simulink model "Dynamic_RLC_system_discrete"  (R2024a)
settings: Solver=FixedStepDiscrete  StartTime=0.0  StopTime=10.0  FixedStep=1e-3  MaxStep=1e-3  RelTol=1e-3
libraries: simulink x1
settings Model: Creator=DELL  LastModifiedBy=DELL

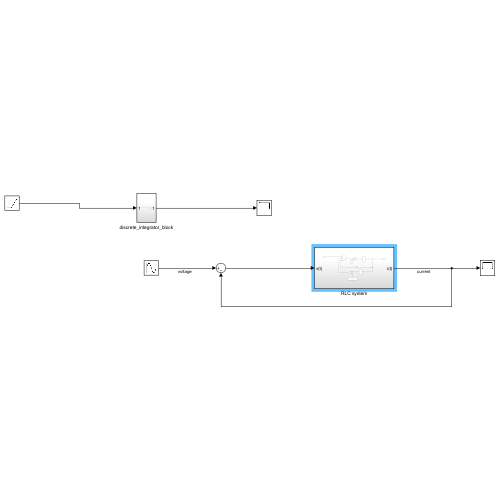
[thumbnail: Simulink's stored preview of the top-level diagram]
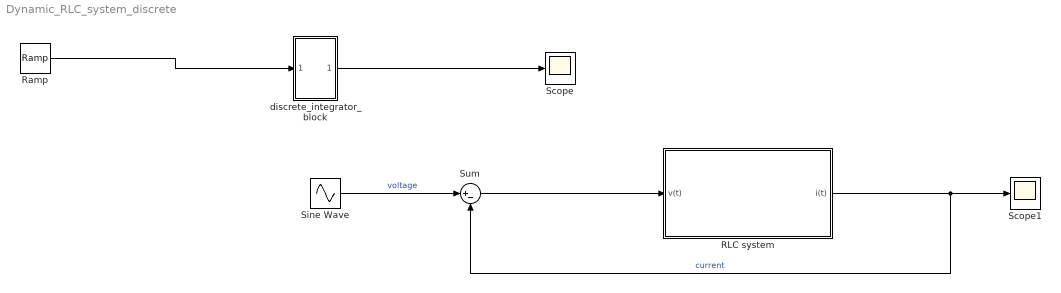
== system Dynamic_RLC_system_discrete ==
  RLC system : Subsystem
  Ramp : simulink/Sources/Ramp  slope=1  start=0  InitialOutput=0
  Scope : Scope
  Scope1 : Scope
  Sine Wave : Sin  Frequency=2000  SampleTime=0
  Sum : Sum  Inputs=|+-
  discrete_integrator_block : Subsystem
  wires:
  Ramp/1 -> discrete_integrator_block/1(In1)
  discrete_integrator_block/1(Out1) -> Scope/1
  Sum/1 -> RLC system/1(v(t))
  Sine Wave/1 -> Sum/1  "voltage"
  RLC system/1(i(t)) -> Sum/2, Scope1/1  "current"

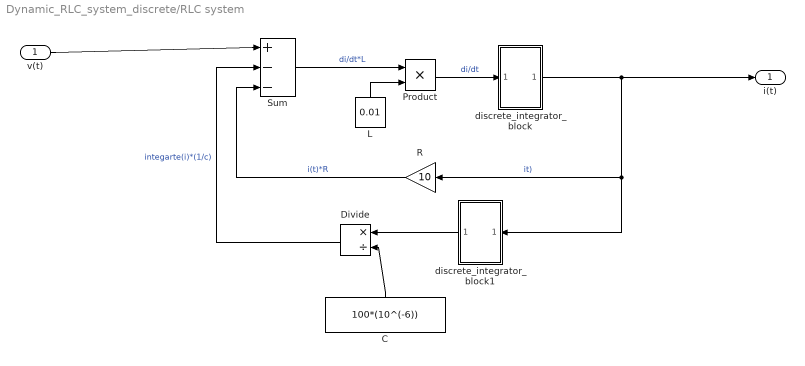
== system Dynamic_RLC_system_discrete/RLC system ==
  v(t) : Inport
  C : Constant  Value=100*(10^(-6))
  Divide : Product  Inputs=*/
  L : Constant  Value=0.01
  Product : Product
  R : Gain  Gain=10
  Sum : Sum  Inputs=|+|-|-
  discrete_integrator_block : Subsystem
  discrete_integrator_block1 : Subsystem
  i(t) : Outport
  wires:
  C/1 -> Divide/2
  L/1 -> Product/2
  discrete_integrator_block/1(Out1) -> i(t)/1, discrete_integrator_block1/1(In1), R/1  "it)"
  Divide/1 -> Sum/2  "integarte(i)*(1/c)"
  discrete_integrator_block1/1(Out1) -> Divide/1
  Product/1 -> discrete_integrator_block/1(In1)  "di/dt"
  Sum/1 -> Product/1  "di/dt*L"
  R/1 -> Sum/3  "i(t)*R"
  v(t)/1 -> Sum/1

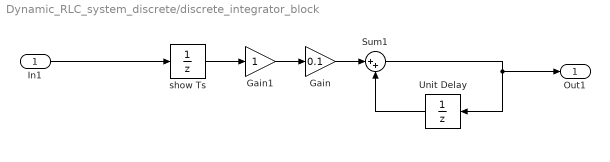
== system Dynamic_RLC_system_discrete/discrete_integrator_block ==
  In1 : Inport
  Gain : Gain  Gain=0.1
  Gain1 : Gain
  Sum1 : Sum  Inputs=|++
  Unit Delay : UnitDelay  SampleTime=-1  HasFrameUpgradeWarning=on
  show Ts : UnitDelay  SampleTime=-1  HasFrameUpgradeWarning=on
  Out1 : Outport
  wires:
  Gain1/1 -> Gain/1
  show Ts/1 -> Gain1/1
  Unit Delay/1 -> Sum1/2
  In1/1 -> show Ts/1
  Sum1/1 -> Out1/1, Unit Delay/1
  Gain/1 -> Sum1/1

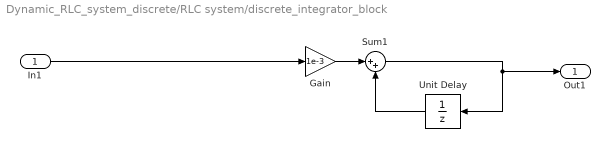
== system Dynamic_RLC_system_discrete/RLC system/discrete_integrator_block ==
  In1 : Inport
  Gain : Gain  Gain=1e-3
  Sum1 : Sum  Inputs=|++
  Unit Delay : UnitDelay  SampleTime=-1  HasFrameUpgradeWarning=on
  Out1 : Outport
  wires:
  In1/1 -> Gain/1
  Unit Delay/1 -> Sum1/2
  Sum1/1 -> Out1/1, Unit Delay/1
  Gain/1 -> Sum1/1

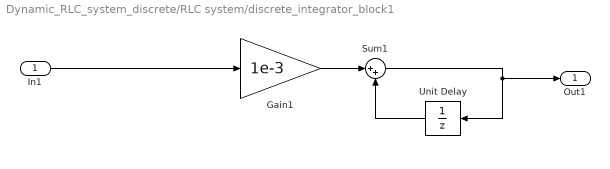
== system Dynamic_RLC_system_discrete/RLC system/discrete_integrator_block1 ==
  In1 : Inport
  Gain1 : Gain  Gain=1e-3
  Sum1 : Sum  Inputs=|++
  Unit Delay : UnitDelay  SampleTime=-1  HasFrameUpgradeWarning=on
  Out1 : Outport
  wires:
  In1/1 -> Gain1/1
  Unit Delay/1 -> Sum1/2
  Sum1/1 -> Out1/1, Unit Delay/1
  Gain1/1 -> Sum1/1
